simulink model "model"  (R2016a)
settings: Solver=FixedStepAuto  StartTime=0.0  StopTime=20  FixedStep=0.01  RelTol=1e-3
settings Model: Creator=Priscilla  LastModifiedBy=Priscilla

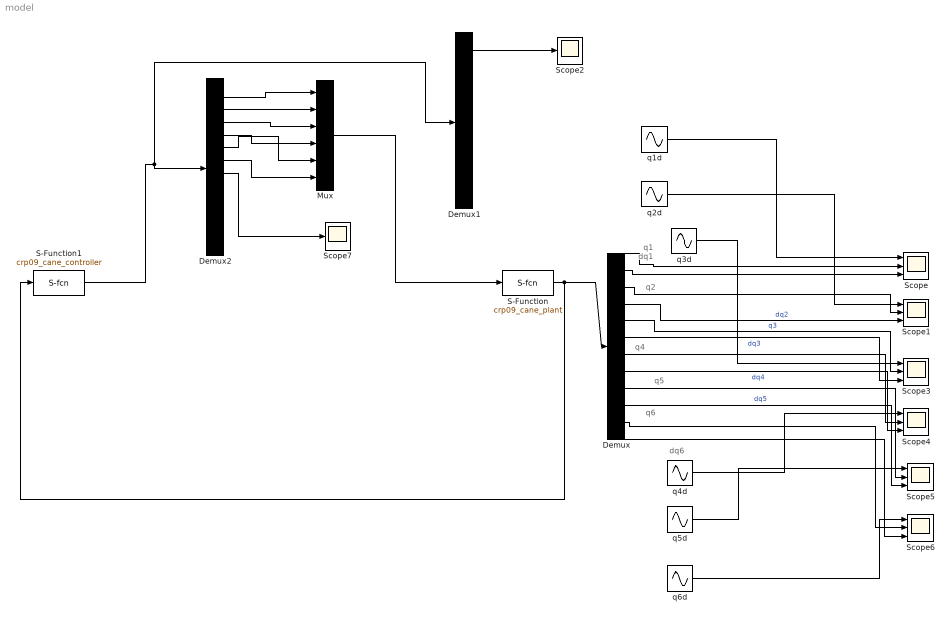
== system model ==
  note: dq6
  note: q6
  note: q5
  note: q4
  note: q2
  note: dq1
  note: q1
  Demux : Demux  Outputs=12
  Demux1 : Demux  Outputs=12
  Demux2 : Demux  Outputs=12
  Mux : Mux  Inputs=6
  S-Function : S-Function  FunctionName=crp09_cane_plant  SFunctionDeploymentMode=off  EnableBusSupport=off
  S-Function1 : S-Function  FunctionName=crp09_cane_controller  SFunctionDeploymentMode=off  EnableBusSupport=off
  Scope{,1,3..6} (6 alike) : Scope  NumInputPorts=3
  Scope2 : Scope
  Scope7 : Scope
  q1d : Sin  SampleTime=0
  q2d : Sin  Frequency=1/2  SampleTime=0
  q3d : Sin  Frequency=1/3  SampleTime=0
  q4d : Sin  Amplitude=0.5  SampleTime=0
  q5d : Sin  Phase=pi/2  SampleTime=0
  q6d : Sin  Frequency=1/2  Phase=pi/2  SampleTime=0
  wires:
  S-Function/1 -> Demux/1, S-Function1/1
  q1d/1 -> Scope/1
  Demux/1 -> Scope/2
  Demux/2 -> Scope/3
  Demux1/1 -> Scope2/1
  Demux/3 -> Scope1/2
  Demux/4 -> Scope1/3  "dq2"
  Demux/5 -> Scope3/2  "q3"
  Demux/6 -> Scope3/3  "dq3"
  Demux/7 -> Scope4/2
  Demux/8 -> Scope4/3  "dq4"
  Demux/9 -> Scope5/2
  Demux/10 -> Scope5/3  "dq5"
  Demux/11 -> Scope6/2
  Demux/12 -> Scope6/3
  q2d/1 -> Scope1/1
  q3d/1 -> Scope3/1
  q4d/1 -> Scope4/1
  q5d/1 -> Scope5/1
  q6d/1 -> Scope6/1
  Demux2/1 -> Mux/1
  Demux2/2 -> Mux/2
  Demux2/3 -> Mux/3
  Demux2/4 -> Mux/4
  Demux2/5 -> Mux/5
  Demux2/6 -> Mux/6
  S-Function1/1 -> Demux1/1, Demux2/1
  Mux/1 -> S-Function/1
  Demux2/7 -> Scope7/1
